simulink model "SingleTrackCANoe"  (R2021b)
settings: Solver=ode1  StartTime=0  StopTime=2  FixedStep=1.0000000000000000e-003  RelTol=1e-3
InitFcn:
  | sampleTime = str2double(get_param(bdroot, 'FixedStep'));
undefined symbols (not defined in the file or in its folder): AccPedalPos, BrakePedalPos, BrakeSwitch, DiscIntNeverNeededParam, DYNA4, EngSpd, IgnitionSwitch, InitialGear, InitialSpeed, IntendedEngTrq, LeftIndicator, MainBrakePress, MaxGear, MDL, MinGear, RefAcc, RefLane, RefLatPos, RefPath, RefPathCurv, RefSpd, RefSpdPreview, RefSpdRetrospect, RightIndicator, SteeringWheelAng, SteeringWheelTrq, UserDefinedRefValue, vm_const
libraries: UtilitiesLibrary x62, simulink x18, WheelSystemModules x14, LongitudinalControllerModules x13, LateralControllerModules x7, AnimationBusselectorModules x5, EnvironmentModules x5, BasicEngineControlModules x5, MiscellaneousControlModules x5, Animation3Modules x4, AuxiliariesModules x4, ReducedTireModules x4
(part 20 of 34)

== system SingleTrackCANoe/SimulationModel/Vehicle/Drivetrain/DrivetrainPhysics/DrivetrainPhysicsOutputs ==
  EngStates : Inport
  ClutchStates : Inport  Port=2
  TransmissionStates : Inport  Port=3
  TransferCase : Inport  Port=4
  FrontDifferentialStates : Inport  Port=5
  RearDifferentialStates : Inport  Port=6
  FrontLeftDifferentialStates : Inport  Port=7
  FrontRightDifferentialStates : Inport  Port=8
  RearLeftDifferentialStates : Inport  Port=9
  RearRightDifferentialStates : Inport  Port=10
  OutputDriveRatio : Inport  Port=11
  Bus Creator : BusCreator  Inputs=1
  Bus Creator4 : BusCreator  Inputs=2
  Bus Selector : BusSelector  OutputSignals=Physics.InSpd[rad/s],Physics.InAcc[rad/s**2]
  Bus Selector2 : BusSelector  OutputSignals=TrqDistributionFac[0_1]
  ClutchOutput : Subsystem
  Create TotalRatio/DrivetrainStates : DrivetrainModules/Create TotalRatio//DrivetrainStates  SystemSampleTime=-1  VariantActivationTime=update diagram  Latency=0  AutoFrameSizeCalculation=off
  DrivetrainPhysicsOutput : Subsystem  Tag=TESIS DYNAware Interface Block  mask{NeedsUpdate=off, SignalInfo=|}
      mask SignalInfo=|
      | {
      |   "Version": "4.6",
      |   "MuxedOutputBusName": "DrivetrainPhysics",
      |   "MuxedInputBusName": "input",
      |   "MuxedInputSelected": false,
      |   "MuxedOutputSelected": true,
      |   "SignalData": [
      |     {
      |       "initialValue": "0.0",
      |       "name": "EngSpd[rad/s]",
      |       "comment": "",
      |       "minString": "",
      |       "maxString": "",
      |       "width": 1,
      |       "dataType": 0,
      |       "signalType": 0,
      |       "createSignal": false,
      |       "outputName": "EngSpd[rad/s]",
      |       "generateSignalAccessBlock": false,
      |       "accessId": "$(parentId).$(blockName).$(outputName)"
      |     },
      |     {
      |       "initialValue": "0.0",
      |       "name": "EngAcc[rad/s**2]",
      |       "comment": "",
      |       "minString": "",
      |       "maxString": "",
      |       "width": 1,
      |       "dataType": 0,
      |       "signalType": 0,
      |       "createSignal": false,
      |       "outputName": "EngAcc[rad/s**2]",
      |       "generateSignalAccessBlock": false,
      |       "accessId": "$(parentId).$(blockName).$(outputName)"
      |     },
      |     {
      |       "initialValue": "0.0",
      |       "name": "Clutch",
      |       "comment": "",
      |       "minString": "",
      |       "maxString": "",
      |       "width": -1,
      |       "dataType": 0,
      |       "signalType": 1,
      |       "createSignal": false,
      |       "outputName": "Clutch",
      |       "generateSignalAccessBlock": false,
      |       "accessId": "$(parentId).$(blockName).$(outputName)"
      |     },
      |     {
      |       "initialValue": "0.0",
      |       "name": "Transmission",
      |       "comment": "",
      |       "minString": "",
      |       "maxString": "",
      |       "width": -1,
      |       "dataType": 0,
      |       "signalType": 1,
      |       "createSignal": false,
      |       "outputName": "Transmission",
      |       "generateSignalAccessBlock": false,
      |       "accessId": "$(parentId).$(blockName).$(outputName)"
      |     },
      |     {
      |       "initialValue": "0.0",
      |       "name": "TransferCase",
      |       "comment": "",
      |       "minString": "",
      |       "maxString": "",
      |       "width": -1,
      |       "dataType": 0,
      |       "signalType": 1,
      |       "createSignal": false,
      |       "outputName": "TransferCase",
      |       "generateSignalAccessBlock": false,
      |       "accessId": "$(parentId).$(blockName).$(outputName)"
      |     },
      |     {
      |       "initialValue": "0.0",
      |       "name": "FrontDifferential",
      |       "comment": "",
      |       "minString": "",
      |       "maxString": "",
      |       "width": -1,
      |       "dataType": 0,
      |       "signalType": 1,
      |       "createSignal": false,
      |       "outputName": "FrontDifferential",
      |       "generateSignalAccessBlock": false,
      |       "accessId": "$(parentId).$(blockName).$(outputName)"
      |     },
      |     {
      |       "initialValue": "0.0",
      |       "name": "FrontLeftShaft",
      |       "comment": "",
      |       "minString": "",
      |       "maxString": "",
      |       "width": -1,
      |       "dataType": 0,
      |       "signalType": 1,
      |       "createSignal": false,
      |       "outputName": "FrontLeftShaft",
      |       "generateSignalAccessBlock": false,
      |       "accessId": "$(parentId).$(blockName).$(outputName)"
      |     },
      |     {
      |       "initialValue": "0.0",
      |       "name": "FrontRightShaft",
      |       "comment": "",
      |       "minString": "",
      |       "maxString": "",
      |       "width": -1,
      |       "dataType": 0,
      |       "signalType": 1,
      |       "createSignal": false,
      |       "outputName": "FrontRightShaft",
      |       "generateSignalAccessBlock": false,
      |       "accessId": "$(parentId).$(blockName).$(outputName)"
      |     },
      |     {
      |       "initialValue": "0.0",
      |       "name": "RearDifferential",
      |       "comment": "",
      |       "minString": "",
      |       "maxString": "",
      |       "width": -1,
      |       "dataType": 0,
      |       "signalType": 1,
      |       "createSignal": false,
      |       "outputName": "RearDifferential",
      |       "generateSignalAccessBlock": false,
      |       "accessId": "$(parentId).$(blockName).$(outputName)"
      |     },
      |     {
      |       "initialValue": "0.0",
      |       "name": "RearLeftShaft",
      |       "comment": "",
      |       "minString": "",
      |       "maxString": "",
      |       "width": -1,
      |       "dataType": 0,
      |       "signalType": 1,
      |       "createSignal": false,
      |       "outputName": "RearLeftShaft",
      |       "generateSignalAccessBlock": false,
      |       "accessId": "$(parentId).$(blockName).$(outputName)"
      |     },
      |     {
      |       "initialValue": "0.0",
      |       "name": "RearRightShaft",
      |       "comment": "",
      |       "minString": "",
      |       "maxString": "",
      |       "width": -1,
      |       "dataType": 0,
      |       "signalType": 1,
      |       "createSignal": false,
      |       "outputName": "RearRightShaft",
      |       "generateSignalAccessBlock": false,
      |       "accessId": "$(parentId).$(blockName).$(outputName)"
      |     },
      |     {
      |       "initialValue": "0.0",
      |       "name": "Rear2LeftShaft",
      |       "comment": "",
      |       "minString": "",
      |       "maxString": "",
      |       "width": -1,
      |       "dataType": 0,
      |       "signalType": 1,
      |       "createSignal": false,
      |       "outputName": "Rear2LeftShaft",
      |       "generateSignalAccessBlock": false,
      |       "accessId": "$(parentId).$(blockName).$(outputName)"
      |     },
      |     {
      |       "initialValue": "0.0",
      |       "name": "Rear2RightShaft",
      |       "comment": "",
      |       "minString": "",
      |       "maxString": "",
      |       "width": -1,
      |       "dataType": 0,
      |       "signalType": 1,
      |       "createSignal": false,
      |       "outputName": "Rear2RightShaft",
      |       "generateSignalAccessBlock": false,
      |       "accessId": "$(parentId).$(blockName).$(outputName)"
      |     },
      |     {
      |       "initialValue": "0.0",
      |       "name": "Rear3LeftShaft",
      |       "comment": "",
      |       "minString": "",
      |       "maxString": "",
      |       "width": -1,
      |       "dataType": 0,
      |       "signalType": 1,
      |       "createSignal": false,
      |       "outputName": "Rear3LeftShaft",
      |       "generateSignalAccessBlock": false,
      |       "accessId": "$(parentId).$(blockName).$(outputName)"
      |     },
      |     {
      |       "initialValue": "0.0",
      |       "name": "Rear3RightShaft",
      |       "comment": "",
      |       "minString": "",
      |       "maxString": "",
      |       "width": -1,
      |       "dataType": 0,
      |       "signalType": 1,
      |       "createSignal": false,
      |       "outputName": "Rear3RightShaft",
      |       "generateSignalAccessBlock": false,
      |       "accessId": "$(parentId).$(blockName).$(outputName)"
      |     },
      |     {
      |       "initialValue": "0.0",
      |       "name": "TotalRatio[-]",
      |       "comment": "",
      |       "minString": "",
      |       "maxString": "",
      |       "width": 1,
      |       "dataType": 0,
      |       "signalType": 0,
      |       "createSignal": false,
      |       "outputName": "TotalRatio[-]",
      |       "generateSignalAccessBlock": false,
      |       "accessId": "$(parentId).$(blockName).$(outputName)"
      |     },
      |     {
      |       "initialValue": "0.0",
      |       "name": "DrivetrainStates",
      |       "comment": "",
      |       "minString": "",
      |       "maxString": "",
      |       "width": -1,
      |       "dataType": 0,
      |       "signalType": 1,
      |       "createSignal": false,
      |       "outputName": "DrivetrainStates",
      |       "generateSignalAccessBlock": false,
      |       "accessId": "$(parentId).$(blockName).$(outputName)"
      |     }
      |   ]
      | }
      mask prompts: NeedsUpdate "Specify, if subsystem content needs to be updated"; SignalInfo "Signal Info (json)"
      mask help: DYNA4 Interface Block Version 4.6
      mask init:
      | blockName = get_param(gcbh, 'Name');
      | parentId = DYNA4.ModelHandling.AccessID.getFromHierarchy(gcbh);
      | TD.InterfaceBlock.ModelCallbacks.GenerateContent(gcb);
      settings: DeleteFcn=TD.InterfaceBlock.ModelCallbacks.CloseGUI( gcbh );  NameChangeFcn=TD.InterfaceBlock.ModelCallbacks.BlockRenamedHandler(gcbh);  OpenFcn=TD.InterfaceBlock.ModelCallbacks.OpenGUI( gcbh );  CloseFcn=TD.InterfaceBlock.ModelCallbacks.CloseGUI( gcbh );
      mask Display:
      | image('InterfaceBlock.png','center');
      | port_label('input',1, 'EngSpd[rad/s]');
      | port_label('input',2, 'EngAcc[rad/s**2]');
      | port_label('input',3, 'Clutch');
      | port_label('input',4, 'Transmission');
      | port_label('input',5, 'TransferCase');
      | port_label('input',6, 'FrontDifferential');
      | port_label('input',7, 'FrontLeftShaft');
      | port_label('input',8, 'FrontRightShaft');
      | port_label('input',9, 'RearDifferential');
      | port_label('input',10, 'RearLeftShaft');
      | port_label('input',11, 'RearRightShaft');
      | port_label('input',12, 'Rear2LeftShaft');
      | port_label('input',13, 'Rear2RightShaft');
      | port_label('input',14, 'Rear3LeftShaft');
      | port_label('input',15, 'Rear3RightShaft');
      | port_label('input',16, 'TotalRatio[-]');
      | port_label('input',17, 'DrivetrainStates');
      | port_label('output',1, 'DrivetrainPhysics');
  FrontDifferentialOutput : Subsystem
  FrontLeftShaftOutput : Subsystem
  FrontRightShaftOutput : Subsystem
  PassThroughRatio : Constant
  Rear2LeftShaftOutput : Subsystem  Tag=TESIS DYNAware Interface Block  mask{NeedsUpdate=off, SignalInfo=|}
      mask SignalInfo=|
      | {
      |   "Version": "4.6",
      |   "MuxedOutputBusName": "Rear2LeftShaft",
      |   "MuxedInputBusName": "input",
      |   "MuxedInputSelected": false,
      |   "MuxedOutputSelected": true,
      |   "SignalData": [
      |     {
      |       "initialValue": "0.0",
      |       "name": "",
      |       "comment": "",
      |       "minString": "",
      |       "maxString": "",
      |       "width": 1,
      |       "dataType": 0,
      |       "signalType": 0,
      |       "createSignal": true,
      |       "outputName": "Trq[Nm]",
      |       "generateSignalAccessBlock": false,
      |       "accessId": "$(parentId).$(blockName).$(outputName)"
      |     },
      |     {
      |       "initialValue": "0.0",
      |       "name": "",
      |       "comment": "",
      |       "minString": "",
      |       "maxString": "",
      |       "width": 1,
      |       "dataType": 0,
      |       "signalType": 0,
      |       "createSignal": true,
      |       "outputName": "RotSpdDifferentialOut[rad/s]",
      |       "generateSignalAccessBlock": false,
      |       "accessId": "$(parentId).$(blockName).$(outputName)"
      |     },
      |     {
      |       "initialValue": "0.0",
      |       "name": "",
      |       "comment": "",
      |       "minString": "",
      |       "maxString": "",
      |       "width": 1,
      |       "dataType": 0,
      |       "signalType": 0,
      |       "createSignal": true,
      |       "outputName": "RotAcc[rad/s**2]",
      |       "generateSignalAccessBlock": false,
      |       "accessId": "$(parentId).$(blockName).$(outputName)"
      |     },
      |     {
      |       "initialValue": "0.0",
      |       "name": "",
      |       "comment": "",
      |       "minString": "",
      |       "maxString": "",
      |       "width": 1,
      |       "dataType": 0,
      |       "signalType": 0,
      |       "createSignal": true,
      |       "outputName": "DerivativeOfTrq_wrt_RotAng[Nm/rad]",
      |       "generateSignalAccessBlock": false,
      |       "accessId": "$(parentId).$(blockName).$(outputName)"
      |     },
      |     {
      |       "initialValue": "0.0",
      |       "name": "",
      |       "comment": "",
      |       "minString": "",
      |       "maxString": "",
      |       "width": 1,
      |       "dataType": 0,
      |       "signalType": 0,
      |       "createSignal": true,
      |       "outputName": "DerivativeOfTrq_wrt_WheelSpd[Nm/(rad/s)]",
      |       "generateSignalAccessBlock": false,
      |       "accessId": "$(parentId).$(blockName).$(outputName)"
      |     },
      |     {
      |       "initialValue": "0.0",
      |       "name": "",
      |       "comment": "",
      |       "minString": "",
      |       "maxString": "",
      |       "width": 1,
      |       "dataType": 0,
      |       "signalType": 0,
      |       "createSignal": true,
      |       "outputName": "AddInrt[kg*m**2]",
      |       "generateSignalAccessBlock": false,
      |       "accessId": "$(parentId).$(blockName).$(outputName)"
      |     },
      |     {
      |       "initialValue": "0.0",
      |       "name": "",
      |       "comment": "",
      |       "minString": "",
      |       "maxString": "",
      |       "width": 1,
      |       "dataType": 0,
      |       "signalType": 0,
      |       "createSignal": true,
      |       "outputName": "FrictionTrq[Nm]",
      |       "generateSignalAccessBlock": false,
      |       "accessId": "$(parentId).$(blockName).$(outputName)"
      |     }
      |   ]
      | }
      mask prompts: NeedsUpdate "Specify, if subsystem content needs to be updated"; SignalInfo "Signal Info (json)"
      mask help: DYNA4 Interface Block Version 4.6
      mask init:
      | blockName = get_param(gcbh, 'Name');
      | parentId = DYNA4.ModelHandling.AccessID.getFromHierarchy(gcbh);
      | TD.InterfaceBlock.ModelCallbacks.GenerateContent(gcb);
      settings: DeleteFcn=TD.InterfaceBlock.ModelCallbacks.CloseGUI( gcbh );  NameChangeFcn=TD.InterfaceBlock.ModelCallbacks.BlockRenamedHandler(gcbh);  OpenFcn=TD.InterfaceBlock.ModelCallbacks.OpenGUI( gcbh );  CloseFcn=TD.InterfaceBlock.ModelCallbacks.CloseGUI( gcbh );
      settings: AttributesFormatString=|
      | Trq[Nm] = 0.0
      | RotSpdDifferentialOut[rad/s] = 0.0
      | RotAcc[rad/s**2] = 0.0
      | DerivativeOfTrq_wrt_RotAng[Nm/rad] = 0.0
      | ...
      mask Display:
      | image('InterfaceBlock.png','center');
      | port_label('output',1, 'Rear2LeftShaft');
  Rear2RightShaftOutput : Subsystem  Tag=TESIS DYNAware Interface Block  mask{NeedsUpdate=off, SignalInfo=|}
      mask SignalInfo=|
      | {
      |   "Version": "4.6",
      |   "MuxedOutputBusName": "Rear2RightShaft",
      |   "MuxedInputBusName": "",
      |   "MuxedInputSelected": false,
      |   "MuxedOutputSelected": true,
      |   "SignalData": [
      |     {
      |       "initialValue": "0.0",
      |       "name": "",
      |       "comment": "",
      |       "minString": "",
      |       "maxString": "",
      |       "width": 1,
      |       "dataType": 0,
      |       "signalType": 0,
      |       "createSignal": true,
      |       "outputName": "Trq[Nm]",
      |       "generateSignalAccessBlock": false,
      |       "accessId": "$(parentId).$(blockName).$(outputName)"
      |     },
      |     {
      |       "initialValue": "0.0",
      |       "name": "",
      |       "comment": "",
      |       "minString": "",
      |       "maxString": "",
      |       "width": 1,
      |       "dataType": 0,
      |       "signalType": 0,
      |       "createSignal": true,
      |       "outputName": "RotSpdDifferentialOut[rad/s]",
      |       "generateSignalAccessBlock": false,
      |       "accessId": "$(parentId).$(blockName).$(outputName)"
      |     },
      |     {
      |       "initialValue": "0.0",
      |       "name": "",
      |       "comment": "",
      |       "minString": "",
      |       "maxString": "",
      |       "width": 1,
      |       "dataType": 0,
      |       "signalType": 0,
      |       "createSignal": true,
      |       "outputName": "RotAcc[rad/s**2]",
      |       "generateSignalAccessBlock": false,
      |       "accessId": "$(parentId).$(blockName).$(outputName)"
      |     },
      |     {
      |       "initialValue": "0.0",
      |       "name": "",
      |       "comment": "",
      |       "minString": "",
      |       "maxString": "",
      |       "width": 1,
      |       "dataType": 0,
      |       "signalType": 0,
      |       "createSignal": true,
      |       "outputName": "DerivativeOfTrq_wrt_RotAng[Nm/rad]",
      |       "generateSignalAccessBlock": false,
      |       "accessId": "$(parentId).$(blockName).$(outputName)"
      |     },
      |     {
      |       "initialValue": "0.0",
      |       "name": "",
      |       "comment": "",
      |       "minString": "",
      |       "maxString": "",
      |       "width": 1,
      |       "dataType": 0,
      |       "signalType": 0,
      |       "createSignal": true,
      |       "outputName": "DerivativeOfTrq_wrt_WheelSpd[Nm/(rad/s)]",
      |       "generateSignalAccessBlock": false,
      |       "accessId": "$(parentId).$(blockName).$(outputName)"
      |     },
      |     {
      |       "initialValue": "0.0",
      |       "name": "",
      |       "comment": "",
      |       "minString": "",
      |       "maxString": "",
      |       "width": 1,
      |       "dataType": 0,
      |       "signalType": 0,
      |       "createSignal": true,
      |       "outputName": "AddInrt[kg*m**2]",
      |       "generateSignalAccessBlock": false,
      |       "accessId": "$(parentId).$(blockName).$(outputName)"
      |     },
      |     {
      |       "initialValue": "0.0",
      |       "name": "",
      |       "comment": "",
      |       "minString": "",
      |       "maxString": "",
      |       "width": 1,
      |       "dataType": 0,
      |       "signalType": 0,
      |       "createSignal": true,
      |       "outputName": "FrictionTrq[Nm]",
      |       "generateSignalAccessBlock": false,
      |       "accessId": "$(parentId).$(blockName).$(outputName)"
      |     }
      |   ]
      | }
      mask prompts: NeedsUpdate "Specify, if subsystem content needs to be updated"; SignalInfo "Signal Info (json)"
      mask help: DYNA4 Interface Block Version 4.6
      mask init:
      | blockName = get_param(gcbh, 'Name');
      | parentId = DYNA4.ModelHandling.AccessID.getFromHierarchy(gcbh);
      | TD.InterfaceBlock.ModelCallbacks.GenerateContent(gcb);
      settings: DeleteFcn=TD.InterfaceBlock.ModelCallbacks.CloseGUI( gcbh );  NameChangeFcn=TD.InterfaceBlock.ModelCallbacks.BlockRenamedHandler(gcbh);  OpenFcn=TD.InterfaceBlock.ModelCallbacks.OpenGUI( gcbh );  CloseFcn=TD.InterfaceBlock.ModelCallbacks.CloseGUI( gcbh );
      settings: AttributesFormatString=|
      | Trq[Nm] = 0.0
      | RotSpdDifferentialOut[rad/s] = 0.0
      | RotAcc[rad/s**2] = 0.0
      | DerivativeOfTrq_wrt_RotAng[Nm/rad] = 0.0
      | ...
      mask Display:
      | image('InterfaceBlock.png','center');
      | port_label('output',1, 'Rear2RightShaft');
  Rear3LeftShaftOutput : Subsystem  Tag=TESIS DYNAware Interface Block  mask{NeedsUpdate=off, SignalInfo=|}
      mask SignalInfo=|
      | {
      |   "Version": "4.6",
      |   "MuxedOutputBusName": "Rear3LeftShaft",
      |   "MuxedInputBusName": "",
      |   "MuxedInputSelected": false,
      |   "MuxedOutputSelected": true,
      |   "SignalData": [
      |     {
      |       "initialValue": "0.0",
      |       "name": "",
      |       "comment": "",
      |       "minString": "",
      |       "maxString": "",
      |       "width": 1,
      |       "dataType": 0,
      |       "signalType": 0,
      |       "createSignal": true,
      |       "outputName": "Trq[Nm]",
      |       "generateSignalAccessBlock": false,
      |       "accessId": "$(parentId).$(blockName).$(outputName)"
      |     },
      |     {
      |       "initialValue": "0.0",
      |       "name": "",
      |       "comment": "",
      |       "minString": "",
      |       "maxString": "",
      |       "width": 1,
      |       "dataType": 0,
      |       "signalType": 0,
      |       "createSignal": true,
      |       "outputName": "RotSpdDifferentialOut[rad/s]",
      |       "generateSignalAccessBlock": false,
      |       "accessId": "$(parentId).$(blockName).$(outputName)"
      |     },
      |     {
      |       "initialValue": "0.0",
      |       "name": "",
      |       "comment": "",
      |       "minString": "",
      |       "maxString": "",
      |       "width": 1,
      |       "dataType": 0,
      |       "signalType": 0,
      |       "createSignal": true,
      |       "outputName": "RotAcc[rad/s**2]",
      |       "generateSignalAccessBlock": false,
      |       "accessId": "$(parentId).$(blockName).$(outputName)"
      |     },
      |     {
      |       "initialValue": "0.0",
      |       "name": "",
      |       "comment": "",
      |       "minString": "",
      |       "maxString": "",
      |       "width": 1,
      |       "dataType": 0,
      |       "signalType": 0,
      |       "createSignal": true,
      |       "outputName": "DerivativeOfTrq_wrt_RotAng[Nm/rad]",
      |       "generateSignalAccessBlock": false,
      |       "accessId": "$(parentId).$(blockName).$(outputName)"
      |     },
      |     {
      |       "initialValue": "0.0",
      |       "name": "",
      |       "comment": "",
      |       "minString": "",
      |       "maxString": "",
      |       "width": 1,
      |       "dataType": 0,
      |       "signalType": 0,
      |       "createSignal": true,
      |       "outputName": "DerivativeOfTrq_wrt_WheelSpd[Nm/(rad/s)]",
      |       "generateSignalAccessBlock": false,
      |       "accessId": "$(parentId).$(blockName).$(outputName)"
      |     },
      |     {
      |       "initialValue": "0.0",
      |       "name": "",
      |       "comment": "",
      |       "minString": "",
      |       "maxString": "",
      |       "width": 1,
      |       "dataType": 0,
      |       "signalType": 0,
      |       "createSignal": true,
      |       "outputName": "AddInrt[kg*m**2]",
      |       "generateSignalAccessBlock": false,
      |       "accessId": "$(parentId).$(blockName).$(outputName)"
      |     },
      |     {
      |       "initialValue": "0.0",
      |       "name": "",
      |       "comment": "",
      |       "minString": "",
      |       "maxString": "",
      |       "width": 1,
      |       "dataType": 0,
      |       "signalType": 0,
      |       "createSignal": true,
      |       "outputName": "FrictionTrq[Nm]",
      |       "generateSignalAccessBlock": false,
      |       "accessId": "$(parentId).$(blockName).$(outputName)"
      |     }
      |   ]
      | }
      mask prompts: NeedsUpdate "Specify, if subsystem content needs to be updated"; SignalInfo "Signal Info (json)"
      mask help: DYNA4 Interface Block Version 4.6
      mask init:
      | blockName = get_param(gcbh, 'Name');
      | parentId = DYNA4.ModelHandling.AccessID.getFromHierarchy(gcbh);
      | TD.InterfaceBlock.ModelCallbacks.GenerateContent(gcb);
      settings: DeleteFcn=TD.InterfaceBlock.ModelCallbacks.CloseGUI( gcbh );  NameChangeFcn=TD.InterfaceBlock.ModelCallbacks.BlockRenamedHandler(gcbh);  OpenFcn=TD.InterfaceBlock.ModelCallbacks.OpenGUI( gcbh );  CloseFcn=TD.InterfaceBlock.ModelCallbacks.CloseGUI( gcbh );
      settings: AttributesFormatString=|
      | Trq[Nm] = 0.0
      | RotSpdDifferentialOut[rad/s] = 0.0
      | RotAcc[rad/s**2] = 0.0
      | DerivativeOfTrq_wrt_RotAng[Nm/rad] = 0.0
      | ...
      mask Display:
      | image('InterfaceBlock.png','center');
      | port_label('output',1, 'Rear3LeftShaft');
  Rear3RightShaftOutput : Subsystem  Tag=TESIS DYNAware Interface Block  mask{NeedsUpdate=off, SignalInfo=|}
      mask SignalInfo=|
      | {
      |   "Version": "4.6",
      |   "MuxedOutputBusName": "Rear3RightShaft",
      |   "MuxedInputBusName": "",
      |   "MuxedInputSelected": false,
      |   "MuxedOutputSelected": true,
      |   "SignalData": [
      |     {
      |       "initialValue": "0.0",
      |       "name": "",
      |       "comment": "",
      |       "minString": "",
      |       "maxString": "",
      |       "width": 1,
      |       "dataType": 0,
      |       "signalType": 0,
      |       "createSignal": true,
      |       "outputName": "Trq[Nm]",
      |       "generateSignalAccessBlock": false,
      |       "accessId": "$(parentId).$(blockName).$(outputName)"
      |     },
      |     {
      |       "initialValue": "0.0",
      |       "name": "",
      |       "comment": "",
      |       "minString": "",
      |       "maxString": "",
      |       "width": 1,
      |       "dataType": 0,
      |       "signalType": 0,
      |       "createSignal": true,
      |       "outputName": "RotSpdDifferentialOut[rad/s]",
      |       "generateSignalAccessBlock": false,
      |       "accessId": "$(parentId).$(blockName).$(outputName)"
      |     },
      |     {
      |       "initialValue": "0.0",
      |       "name": "",
      |       "comment": "",
      |       "minString": "",
      |       "maxString": "",
      |       "width": 1,
      |       "dataType": 0,
      |       "signalType": 0,
      |       "createSignal": true,
      |       "outputName": "RotAcc[rad/s**2]",
      |       "generateSignalAccessBlock": false,
      |       "accessId": "$(parentId).$(blockName).$(outputName)"
      |     },
      |     {
      |       "initialValue": "0.0",
      |       "name": "",
      |       "comment": "",
      |       "minString": "",
      |       "maxString": "",
      |       "width": 1,
      |       "dataType": 0,
      |       "signalType": 0,
      |       "createSignal": true,
      |       "outputName": "DerivativeOfTrq_wrt_RotAng[Nm/rad]",
      |       "generateSignalAccessBlock": false,
      |       "accessId": "$(parentId).$(blockName).$(outputName)"
      |     },
      |     {
      |       "initialValue": "0.0",
      |       "name": "",
      |       "comment": "",
      |       "minString": "",
      |       "maxString": "",
      |       "width": 1,
      |       "dataType": 0,
      |       "signalType": 0,
      |       "createSignal": true,
      |       "outputName": "DerivativeOfTrq_wrt_WheelSpd[Nm/(rad/s)]",
      |       "generateSignalAccessBlock": false,
      |       "accessId": "$(parentId).$(blockName).$(outputName)"
      |     },
      |     {
      |       "initialValue": "0.0",
      |       "name": "",
      |       "comment": "",
      |       "minString": "",
      |       "maxString": "",
      |       "width": 1,
      |       "dataType": 0,
      |       "signalType": 0,
      |       "createSignal": true,
      |       "outputName": "AddInrt[kg*m**2]",
      |       "generateSignalAccessBlock": false,
      |       "accessId": "$(parentId).$(blockName).$(outputName)"
      |     },
      |     {
      |       "initialValue": "0.0",
      |       "name": "",
      |       "comment": "",
      |       "minString": "",
      |       "maxString": "",
      |       "width": 1,
      |       "dataType": 0,
      |       "signalType": 0,
      |       "createSignal": true,
      |       "outputName": "FrictionTrq[Nm]",
      |       "generateSignalAccessBlock": false,
      |       "accessId": "$(parentId).$(blockName).$(outputName)"
      |     }
      |   ]
      | }
      mask prompts: NeedsUpdate "Specify, if subsystem content needs to be updated"; SignalInfo "Signal Info (json)"
      mask help: DYNA4 Interface Block Version 4.6
      mask init:
      | blockName = get_param(gcbh, 'Name');
      | parentId = DYNA4.ModelHandling.AccessID.getFromHierarchy(gcbh);
      | TD.InterfaceBlock.ModelCallbacks.GenerateContent(gcb);
      settings: DeleteFcn=TD.InterfaceBlock.ModelCallbacks.CloseGUI( gcbh );  NameChangeFcn=TD.InterfaceBlock.ModelCallbacks.BlockRenamedHandler(gcbh);  OpenFcn=TD.InterfaceBlock.ModelCallbacks.OpenGUI( gcbh );  CloseFcn=TD.InterfaceBlock.ModelCallbacks.CloseGUI( gcbh );
      settings: AttributesFormatString=|
      | Trq[Nm] = 0.0
      | RotSpdDifferentialOut[rad/s] = 0.0
      | RotAcc[rad/s**2] = 0.0
      | DerivativeOfTrq_wrt_RotAng[Nm/rad] = 0.0
      | ...
      mask Display:
      | image('InterfaceBlock.png','center');
      | port_label('output',1, 'Rear3RightShaft');
  RearDifferentialOutput : Subsystem
  RearLeftShaftOutput : Subsystem
  RearRightShaftOutput : Subsystem
  Terminator : Terminator
  TotalRatio : Subsystem
  TransferCaseOutput : Subsystem
  TransmissionOutput : Subsystem
  DrivetrainPhysics : Outport  VectorParamsAs1DForOutWhenUnconnected=off
  wires:
  TransferCase/1 -> Bus Selector2/1, TransferCaseOutput/1(TransferCaseStates)
  TransmissionStates/1 -> TransmissionOutput/1(TransmissionStates), Create TotalRatio/DrivetrainStates/1, TotalRatio/1(TransmissionStates)
  EngStates/1 -> Bus Selector/1
  DrivetrainPhysicsOutput/1(DrivetrainPhysics___UNIQUE_1) -> DrivetrainPhysics/1
  ClutchOutput/1(Clutch) -> DrivetrainPhysicsOutput/3(Clutch___UNIQUE_1)
  TransmissionOutput/1(Transmission) -> DrivetrainPhysicsOutput/4(Transmission___UNIQUE_1)
  FrontLeftShaftOutput/1(FrontLeftShaft) -> DrivetrainPhysicsOutput/7(FrontLeftShaft___UNIQUE_1)
  FrontRightShaftOutput/1(FrontRightShaft) -> DrivetrainPhysicsOutput/8(FrontRightShaft___UNIQUE_1)
  RearRightShaftOutput/1(RearRightShaft) -> DrivetrainPhysicsOutput/11(RearRightShaft___UNIQUE_1)
  Rear2LeftShaftOutput/1(Rear2LeftShaft___UNIQUE_1) -> DrivetrainPhysicsOutput/12(Rear2LeftShaft___UNIQUE_1)
  Rear2RightShaftOutput/1(Rear2RightShaft___UNIQUE_1) -> DrivetrainPhysicsOutput/13(Rear2RightShaft___UNIQUE_1)
  Rear3LeftShaftOutput/1(Rear3LeftShaft___UNIQUE_1) -> DrivetrainPhysicsOutput/14(Rear3LeftShaft___UNIQUE_1)
  Rear3RightShaftOutput/1(Rear3RightShaft___UNIQUE_1) -> DrivetrainPhysicsOutput/15(Rear3RightShaft___UNIQUE_1)
  TotalRatio/1(TotalRatio) -> DrivetrainPhysicsOutput/16(TotalRatio[-]___UNIQUE_1)
  ClutchStates/1 -> ClutchOutput/1(ClutchStates)
  RearLeftShaftOutput/1(RearLeftShaft) -> DrivetrainPhysicsOutput/10(RearLeftShaft___UNIQUE_1)
  FrontDifferentialStates/1 -> FrontDifferentialOutput/1(FrontDifferentialStates)
  RearDifferentialStates/1 -> RearDifferentialOutput/1(RearDifferentialStates)
  RearLeftDifferentialStates/1 -> RearLeftShaftOutput/1(In1)
  RearRightDifferentialStates/1 -> RearRightShaftOutput/1(In1)
  FrontLeftDifferentialStates/1 -> FrontLeftShaftOutput/1(In1)
  FrontRightDifferentialStates/1 -> FrontRightShaftOutput/1(In1)
  Bus Selector/1 -> DrivetrainPhysicsOutput/1(EngSpd[rad/s]___UNIQUE_1)  "<InSpd[rad/s]>"
  Bus Selector/2 -> DrivetrainPhysicsOutput/2(EngAcc[rad/s**2]___UNIQUE_1)  "<InAcc[rad/s**2]>"
  TransferCaseOutput/1(TransferCase) -> DrivetrainPhysicsOutput/5(TransferCase___UNIQUE_1)
  FrontDifferentialOutput/1(FrontDifferential) -> DrivetrainPhysicsOutput/6(FrontDifferential___UNIQUE_1)
  RearDifferentialOutput/1(RearDifferential) -> DrivetrainPhysicsOutput/9(RearDifferential___UNIQUE_1)
  OutputDriveRatio/1 -> TotalRatio/2(OutputDriveRatio)
  Create TotalRatio/DrivetrainStates/1 -> Terminator/1
  Create TotalRatio/DrivetrainStates/2 -> DrivetrainPhysicsOutput/17(DrivetrainStates___UNIQUE_1)
  Bus Creator/1 -> Create TotalRatio/DrivetrainStates/2  "Info"
  PassThroughRatio/1 -> Bus Creator/1, Bus Creator4/1  "Ratio[-]"
  Bus Selector2/1 -> Bus Creator4/2  "<TrqDistributionFac[0_1]>"
  Bus Creator4/1 -> Create TotalRatio/DrivetrainStates/3, Create TotalRatio/DrivetrainStates/4, Create TotalRatio/DrivetrainStates/5  "Info"

== system SingleTrackCANoe/SimulationModel/Vehicle/Drivetrain/DrivetrainPhysics/DynaComponentInfo ==

== system SingleTrackCANoe/SimulationModel/Vehicle/Engine/EngineControlUnit/DynaComponentInfo ==

== system SingleTrackCANoe/SimulationModel/Vehicle/Engine/EngineControlUnit/EngineControlUnitOutput ==
  StarterSwitch[0;1]___UNIQUE_1 : Inport  Description=|  PortDimensions=[1]
      | <name>StarterSwitch[0;1]</name>
      | <comment>Engine starter switch</comment>
  EngRunPermission[0;1]___UNIQUE_1 : Inport  Description=|  Port=2  PortDimensions=[1]
      | <name>EngRunPermission[0;1]</name>
      | <comment>Switch indicating a engine stop due to start stop function or ignition off</comment>
  EngLoadSignal[0_1]___UNIQUE_1 : Inport  Description=|  Port=3  PortDimensions=[1]
      | <name>EngLoadSignal[0_1]</name>
      | <comment>Engine load signal</comment>
  EngIdleSpd[rad/s]___UNIQUE_1 : Inport  Description=|  Port=4  PortDimensions=[1]
      | <name>EngIdleSpd[rad/s]</name>
      | <comment>Engine idle speed</comment>
  EngFuelCutoff[0;1]___UNIQUE_1 : Inport  Description=|  Port=5  PortDimensions=[1]
      | <name>EngFuelCutoff[0;1]</name>
      | <comment>Logical signal which is true if fuel mass flow is stopped</comment>
  MaxEngSpd[rad/s]___UNIQUE_1 : Inport  Description=|  Port=6  PortDimensions=[1]
      | <name>MaxEngSpd[rad/s]</name>
      | <comment>Maximum allowed engine speed, threshold for fuel cut off</comment>
  UpperEngTrqSwitch[0;2]___UNIQUE_1 : Inport  Description=|  Port=7  PortDimensions=[1]
      | <name>UpperEngTrqSwitch[0;2]</name>
      | <comment>Switch indicating how the upper engine torque should be restricted (0: off, 1: slow, 2: fast)</comment>
  UpperEngTrqLimit[Nm]___UNIQUE_1 : Inport  Description=|  Port=8  PortDimensions=[1]
      | <name>UpperEngTrqLimit[Nm]</name>
      | <comment>Upper limit for the engine torque</comment>
  LowerEngTrqSwitch[0;2]___UNIQUE_1 : Inport  Description=|  Port=9  PortDimensions=[1]
      | <name>LowerEngTrqSwitch[0;2]</name>
      | <comment>Switch indicating how the lower engine torque should be restricted (0: off, 1: slow, 2: fast)</comment>
  LowerEngTrqLimit[Nm]___UNIQUE_1 : Inport  Description=|  Port=10  PortDimensions=[1]
      | <name>LowerEngTrqLimit[Nm]</name>
      | <comment>Lower limit for the engine torque</comment>
  __TDD__EngineControlUnit.EngFuelCutoff[0;1] : Demux  Outputs=[1]
  __TDD__EngineControlUnit.EngIdleSpd[rad/s] : Demux  Outputs=[1]
  __TDD__EngineControlUnit.EngLoadSignal[0_1] : Demux  Outputs=[1]
  __TDD__EngineControlUnit.EngRunPermission[0;1] : Demux  Outputs=[1]
  __TDD__EngineControlUnit.LowerEngTrqLimit[Nm] : Demux  Outputs=[1]
  __TDD__EngineControlUnit.LowerEngTrqSwitch[0;2] : Demux  Outputs=[1]
  __TDD__EngineControlUnit.MaxEngSpd[rad/s] : Demux  Outputs=[1]
  __TDD__EngineControlUnit.StarterSwitch[0;1] : Demux  Outputs=[1]
  __TDD__EngineControlUnit.UpperEngTrqLimit[Nm] : Demux  Outputs=[1]
  __TDD__EngineControlUnit.UpperEngTrqSwitch[0;2] : Demux  Outputs=[1]
  __TDO__EngineControlUnit : BusCreator  Inputs=10
  EngineControlUnit___UNIQUE_1 : Outport  Description=|  PortDimensions=[10]  VectorParamsAs1DForOutWhenUnconnected=off
      | <name>StarterSwitch[0;1]</name>
      | <comment>Engine starter switch</comment>
  wires:
  __TDO__EngineControlUnit/1 -> EngineControlUnit___UNIQUE_1/1  "EngineControlUnit"
  __TDD__EngineControlUnit.LowerEngTrqLimit[Nm]/1 -> __TDO__EngineControlUnit/10  "LowerEngTrqLimit[Nm]"
  LowerEngTrqLimit[Nm]___UNIQUE_1/1 -> __TDD__EngineControlUnit.LowerEngTrqLimit[Nm]/1
  __TDD__EngineControlUnit.LowerEngTrqSwitch[0;2]/1 -> __TDO__EngineControlUnit/9  "LowerEngTrqSwitch[0;2]"
  LowerEngTrqSwitch[0;2]___UNIQUE_1/1 -> __TDD__EngineControlUnit.LowerEngTrqSwitch[0;2]/1
  __TDD__EngineControlUnit.UpperEngTrqLimit[Nm]/1 -> __TDO__EngineControlUnit/8  "UpperEngTrqLimit[Nm]"
  UpperEngTrqLimit[Nm]___UNIQUE_1/1 -> __TDD__EngineControlUnit.UpperEngTrqLimit[Nm]/1
  __TDD__EngineControlUnit.UpperEngTrqSwitch[0;2]/1 -> __TDO__EngineControlUnit/7  "UpperEngTrqSwitch[0;2]"
  UpperEngTrqSwitch[0;2]___UNIQUE_1/1 -> __TDD__EngineControlUnit.UpperEngTrqSwitch[0;2]/1
  __TDD__EngineControlUnit.MaxEngSpd[rad/s]/1 -> __TDO__EngineControlUnit/6  "MaxEngSpd[rad/s]"
  MaxEngSpd[rad/s]___UNIQUE_1/1 -> __TDD__EngineControlUnit.MaxEngSpd[rad/s]/1
  __TDD__EngineControlUnit.EngFuelCutoff[0;1]/1 -> __TDO__EngineControlUnit/5  "EngFuelCutoff[0;1]"
  EngFuelCutoff[0;1]___UNIQUE_1/1 -> __TDD__EngineControlUnit.EngFuelCutoff[0;1]/1
  __TDD__EngineControlUnit.EngIdleSpd[rad/s]/1 -> __TDO__EngineControlUnit/4  "EngIdleSpd[rad/s]"
  EngIdleSpd[rad/s]___UNIQUE_1/1 -> __TDD__EngineControlUnit.EngIdleSpd[rad/s]/1
  __TDD__EngineControlUnit.EngLoadSignal[0_1]/1 -> __TDO__EngineControlUnit/3  "EngLoadSignal[0_1]"
  EngLoadSignal[0_1]___UNIQUE_1/1 -> __TDD__EngineControlUnit.EngLoadSignal[0_1]/1
  __TDD__EngineControlUnit.EngRunPermission[0;1]/1 -> __TDO__EngineControlUnit/2  "EngRunPermission[0;1]"
  EngRunPermission[0;1]___UNIQUE_1/1 -> __TDD__EngineControlUnit.EngRunPermission[0;1]/1
  __TDD__EngineControlUnit.StarterSwitch[0;1]/1 -> __TDO__EngineControlUnit/1  "StarterSwitch[0;1]"
  StarterSwitch[0;1]___UNIQUE_1/1 -> __TDD__EngineControlUnit.StarterSwitch[0;1]/1

== system SingleTrackCANoe/SimulationModel/Vehicle/Engine/EngineControlUnit/InputFromCTRL ==
  fromCTRL : Inport
  TDBusSelector : BusSelector  OutputSignals=CTRL.LongitudinalControl.IgnitionSwitch[0;3],CTRL.LongitudinalControl.EngRunPermission[0;1],CTRL.LongitudinalControl.AccPedalPos[0_1],CTRL.LongitudinalControl.IntendedEngTrq[Nm],CTRL.LongitudinalControl.IntendedEngTrqActive[0;1],CTRL.LongitudinalControl.ClutchPos[0_1]
  __TDD__AccPedalPos[0_1] : Demux  Outputs=1
  __TDD__ClutchPos[0_1] : Demux  Outputs=[1]
  __TDD__EngRunPermission[0;1] : Demux  Outputs=[1]
  __TDD__IgnitionSwitch[0;3] : Demux  Outputs=[1]
  __TDD__IntendedEngTrqActive[0;1] : Demux  Outputs=[1]
  __TDD__IntendedEngTrq[Nm] : Demux  Outputs=[1]
  IgnitionSwitch[0;3]___UNIQUE_1 : Outport  Description=|  PortDimensions=[1]  VectorParamsAs1DForOutWhenUnconnected=off
      | <name>CTRL.LongitudinalControl.IgnitionSwitch[0;3]</name>
      | <comment>Ignition signal with four signal states: 0 - ignition off + consumer off + starter off, 1 - ignition off + consumer on + starter off, 2 - ignition on + consumer on + starter off, 3 - ignition on + consumer on  + starter on</comment>
  EngRunPermission[0;1]___UNIQUE_1 : Outport  Description=|  Port=2  PortDimensions=[1]  VectorParamsAs1DForOutWhenUnconnected=off
      | <name>CTRL.LongitudinalControl.EngRunPermission[0;1]</name>
      | <comment></comment>
  AccPedalPos[0_1]___UNIQUE_1 : Outport  Description=|  Port=3  VectorParamsAs1DForOutWhenUnconnected=off
      | <name>CTRL.LongitudinalControl.AccPedalPos[0_1]</name>
      | <comment></comment>
  IntendedEngTrq[Nm]___UNIQUE_1 : Outport  Description=|  Port=4  PortDimensions=[1]  VectorParamsAs1DForOutWhenUnconnected=off
      | <name>CTRL.LongitudinalControl.IntendedEngTrq[Nm]</name>
      | <comment></comment>
  IntendedEngTrqActive[0;1]___UNIQUE_1 : Outport  Description=|  Port=5  PortDimensions=[1]  VectorParamsAs1DForOutWhenUnconnected=off
      | <name>CTRL.LongitudinalControl.IntendedEngTrqActive[0;1]</name>
      | <comment></comment>
  ClutchPos[0_1]___UNIQUE_1 : Outport  Description=|  Port=6  PortDimensions=[1]  VectorParamsAs1DForOutWhenUnconnected=off
      | <name>CTRL.LongitudinalControl.ClutchPos[0_1]</name>
      | <comment>Clutch position</comment>
  wires:
  __TDD__ClutchPos[0_1]/1 -> ClutchPos[0_1]___UNIQUE_1/1  "ClutchPos[0_1]"
  __TDD__IntendedEngTrqActive[0;1]/1 -> IntendedEngTrqActive[0;1]___UNIQUE_1/1  "IntendedEngTrqActive[0;1]"
  __TDD__IntendedEngTrq[Nm]/1 -> IntendedEngTrq[Nm]___UNIQUE_1/1  "IntendedEngTrq[Nm]"
  __TDD__AccPedalPos[0_1]/1 -> AccPedalPos[0_1]___UNIQUE_1/1  "AccPedalPos[0_1]"
  __TDD__EngRunPermission[0;1]/1 -> EngRunPermission[0;1]___UNIQUE_1/1  "EngRunPermission[0;1]"
  __TDD__IgnitionSwitch[0;3]/1 -> IgnitionSwitch[0;3]___UNIQUE_1/1  "IgnitionSwitch[0;3]"
  TDBusSelector/6 -> __TDD__ClutchPos[0_1]/1  "<ClutchPos[0_1]>"
  TDBusSelector/5 -> __TDD__IntendedEngTrqActive[0;1]/1  "<IntendedEngTrqActive[0;1]>"
  TDBusSelector/4 -> __TDD__IntendedEngTrq[Nm]/1  "<IntendedEngTrq[Nm]>"
  TDBusSelector/3 -> __TDD__AccPedalPos[0_1]/1  "<AccPedalPos[0_1]>"
  TDBusSelector/2 -> __TDD__EngRunPermission[0;1]/1  "<EngRunPermission[0;1]>"
  TDBusSelector/1 -> __TDD__IgnitionSwitch[0;3]/1  "<IgnitionSwitch[0;3]>"
  fromCTRL/1 -> TDBusSelector/1

== system SingleTrackCANoe/SimulationModel/Vehicle/Engine/EngineControlUnit/InputFromCTRL1 ==
  fromCTRL : Inport
  TDBusSelector : BusSelector  OutputSignals=CTRL.LongitudinalControl.ASRRequestSwitch[0;2],CTRL.LongitudinalControl.ASRTrq[Nm],CTRL.LongitudinalControl.MSRRequestSwitch[0;2],CTRL.LongitudinalControl.MSRTrq[Nm]
  __TDD__ASRRequestSwitch[0;2] : Demux  Outputs=1
  __TDD__ASRTrq[Nm] : Demux  Outputs=1
  __TDD__MSRRequestSwitch[0;2] : Demux  Outputs=1
  __TDD__MSRTrq[Nm] : Demux  Outputs=1
  ASRRequestSwitch[0;2]___UNIQUE_1 : Outport  Description=|  VectorParamsAs1DForOutWhenUnconnected=off
      | <name>CTRL.LongitudinalControl.ASRRequestSwitch[0;2]</name>
      | <comment></comment>
  ASRTrq[Nm]___UNIQUE_1 : Outport  Description=|  Port=2  VectorParamsAs1DForOutWhenUnconnected=off
      | <name>CTRL.LongitudinalControl.ASRTrq[Nm]</name>
      | <comment></comment>
  MSRRequestSwitch[0;2]___UNIQUE_1 : Outport  Description=|  Port=3  VectorParamsAs1DForOutWhenUnconnected=off
      | <name>CTRL.LongitudinalControl.MSRRequestSwitch[0;2]</name>
      | <comment></comment>
  MSRTrq[Nm]___UNIQUE_1 : Outport  Description=|  Port=4  VectorParamsAs1DForOutWhenUnconnected=off
      | <name>CTRL.LongitudinalControl.MSRTrq[Nm]</name>
      | <comment></comment>
  wires:
  __TDD__MSRTrq[Nm]/1 -> MSRTrq[Nm]___UNIQUE_1/1  "MSRTrq[Nm]"
  __TDD__MSRRequestSwitch[0;2]/1 -> MSRRequestSwitch[0;2]___UNIQUE_1/1  "MSRRequestSwitch[0;2]"
  __TDD__ASRTrq[Nm]/1 -> ASRTrq[Nm]___UNIQUE_1/1  "ASRTrq[Nm]"
  __TDD__ASRRequestSwitch[0;2]/1 -> ASRRequestSwitch[0;2]___UNIQUE_1/1  "ASRRequestSwitch[0;2]"
  TDBusSelector/4 -> __TDD__MSRTrq[Nm]/1  "<MSRTrq[Nm]>"
  TDBusSelector/3 -> __TDD__MSRRequestSwitch[0;2]/1  "<MSRRequestSwitch[0;2]>"
  TDBusSelector/2 -> __TDD__ASRTrq[Nm]/1  "<ASRTrq[Nm]>"
  TDBusSelector/1 -> __TDD__ASRRequestSwitch[0;2]/1  "<ASRRequestSwitch[0;2]>"
  fromCTRL/1 -> TDBusSelector/1

== system SingleTrackCANoe/SimulationModel/Vehicle/Engine/EngineControlUnit/InputFromChassis ==
  fromChassis : Inport
  TDBusSelector : BusSelector  OutputSignals=VehicleBody.AbsVel[m/s]
  __TDD__AbsVel[m/s] : Demux  Outputs=1
  AbsVel[m/s]___UNIQUE_1 : Outport  Description=|  VectorParamsAs1DForOutWhenUnconnected=off
      | <name>VehicleBody.AbsVel[m/s]</name>
      | <comment></comment>
  wires:
  __TDD__AbsVel[m/s]/1 -> AbsVel[m/s]___UNIQUE_1/1  "AbsVel[m/s]"
  TDBusSelector/1 -> __TDD__AbsVel[m/s]/1  "<AbsVel[m/s]>"
  fromChassis/1 -> TDBusSelector/1

== system SingleTrackCANoe/SimulationModel/Vehicle/Engine/EngineControlUnit/InputFromDrivetrain ==
  fromDrivetrain : Inport
  TDBusSelector : BusSelector  OutputSignals=DrivetrainPhysics.Transmission.Gear[-4;20],DrivetrainPhysics.EngSpd[rad/s]
  __TDD__EngSpd[rad/s] : Demux  Outputs=1
  __TDD__Gear[-4;20] : Demux  Outputs=1
  Gear[-4;20] : Outport  Description=|  VectorParamsAs1DForOutWhenUnconnected=off
      | <name>DrivetrainPhysics.Transmission.Gear[-4;20]</name>
      | <comment></comment>
  EngSpd[rad/s] : Outport  Description=|  Port=2  VectorParamsAs1DForOutWhenUnconnected=off
      | <name>DrivetrainPhysics.EngSpd[rad/s]</name>
      | <comment></comment>
  wires:
  __TDD__EngSpd[rad/s]/1 -> EngSpd[rad/s]/1  "EngSpd[rad/s]"
  __TDD__Gear[-4;20]/1 -> Gear[-4;20]/1  "Gear[-4;20]"
  TDBusSelector/2 -> __TDD__EngSpd[rad/s]/1  "<EngSpd[rad/s]>"
  TDBusSelector/1 -> __TDD__Gear[-4;20]/1  "<Gear[-4;20]>"
  fromDrivetrain/1 -> TDBusSelector/1

== system SingleTrackCANoe/SimulationModel/Vehicle/Engine/EngineControlUnit/InputFromEnginePhysics ==
  fromEnginePhysics : Inport
  TDBusSelector : BusSelector  OutputSignals=Mechanics.EngTrq[Nm],Mechanics.UnrestrictedEngTrq[Nm],Mechanics.MeanEngFrictionTrq[Nm],Mechanics.MeanEngMaxTrq[Nm]
  __TDD__EngTrq[Nm] : Demux  Outputs=[1]
  __TDD__MeanEngFrictionTrq[Nm] : Demux  Outputs=1
  __TDD__MeanEngMaxTrq[Nm] : Demux  Outputs=1
  __TDD__UnrestrictedEngTrq[Nm] : Demux  Outputs=[1]
  EngTrq[Nm]___UNIQUE_1 : Outport  Description=|  PortDimensions=[1]  VectorParamsAs1DForOutWhenUnconnected=off
      | <name>Mechanics.EngTrq[Nm]</name>
      | <comment>Engine torque</comment>
  UnrestrictedEngTrq[Nm]___UNIQUE_1 : Outport  Description=|  Port=2  PortDimensions=[1]  VectorParamsAs1DForOutWhenUnconnected=off
      | <name>Mechanics.UnrestrictedEngTrq[Nm]</name>
      | <comment>Unrestricted engine torque</comment>
  MeanEngFrictionTrq[Nm]___UNIQUE_1 : Outport  Description=|  Port=3  VectorParamsAs1DForOutWhenUnconnected=off
      | <name>Mechanics.MeanEngFrictionTrq[Nm]</name>
      | <comment></comment>
  MeanEngMaxTrq[Nm]___UNIQUE_1 : Outport  Description=|  Port=4  VectorParamsAs1DForOutWhenUnconnected=off
      | <name>Mechanics.MeanEngMaxTrq[Nm]</name>
      | <comment></comment>
  wires:
  __TDD__MeanEngMaxTrq[Nm]/1 -> MeanEngMaxTrq[Nm]___UNIQUE_1/1  "MeanEngMaxTrq[Nm]"
  __TDD__MeanEngFrictionTrq[Nm]/1 -> MeanEngFrictionTrq[Nm]___UNIQUE_1/1  "MeanEngFrictionTrq[Nm]"
  __TDD__UnrestrictedEngTrq[Nm]/1 -> UnrestrictedEngTrq[Nm]___UNIQUE_1/1  "UnrestrictedEngTrq[Nm]"
  __TDD__EngTrq[Nm]/1 -> EngTrq[Nm]___UNIQUE_1/1  "EngTrq[Nm]"
  TDBusSelector/4 -> __TDD__MeanEngMaxTrq[Nm]/1  "<MeanEngMaxTrq[Nm]>"
  TDBusSelector/3 -> __TDD__MeanEngFrictionTrq[Nm]/1  "<MeanEngFrictionTrq[Nm]>"
  TDBusSelector/2 -> __TDD__UnrestrictedEngTrq[Nm]/1  "<UnrestrictedEngTrq[Nm]>"
  TDBusSelector/1 -> __TDD__EngTrq[Nm]/1  "<EngTrq[Nm]>"
  fromEnginePhysics/1 -> TDBusSelector/1

== system SingleTrackCANoe/SimulationModel/Vehicle/Engine/EnginePhysics/DynaComponentInfo ==

== system SingleTrackCANoe/SimulationModel/Vehicle/Engine/EnginePhysics/EnginePhysicsOutput ==
  Mechanics___UNIQUE_1 : Inport  Description=|
      | <name>Mechanics</name>
      | <comment></comment>
  ValidityStatus___UNIQUE_1 : Inport  Description=|  Port=2
      | <name>ValidityStatus</name>
      | <comment></comment>
  FuelSystem___UNIQUE_1 : Inport  Description=|  Port=3
      | <name>FuelSystem</name>
      | <comment></comment>
  __TDO__EnginePhysics : BusCreator  Inputs=3
  EnginePhysics___UNIQUE_1 : Outport  Description=|  VectorParamsAs1DForOutWhenUnconnected=off
      | <name>Mechanics</name>
      | <comment></comment>
  wires:
  __TDO__EnginePhysics/1 -> EnginePhysics___UNIQUE_1/1  "EnginePhysics"
  FuelSystem___UNIQUE_1/1 -> __TDO__EnginePhysics/3  "FuelSystem"
  ValidityStatus___UNIQUE_1/1 -> __TDO__EnginePhysics/2  "ValidityStatus"
  Mechanics___UNIQUE_1/1 -> __TDO__EnginePhysics/1  "Mechanics"

== system SingleTrackCANoe/SimulationModel/Vehicle/Engine/EnginePhysics/FuelSystemOutput ==
  FuelMassFlow[kg/s]___UNIQUE_1 : Inport  Description=|  PortDimensions=[1]
      | <name>FuelMassFlow[kg/s]</name>
      | <comment></comment>
  FuelMass[kg]___UNIQUE_1 : Inport  Description=|  Port=2  PortDimensions=[1]
      | <name>FuelMass[kg]</name>
      | <comment></comment>
  CurrFuelConsumEu[l/100km]___UNIQUE_1 : Inport  Description=|  Port=3  PortDimensions=[1]
      | <name>CurrFuelConsumEu[l/100km]</name>
      | <comment></comment>
  CurrFuelConsumUs[mpg]___UNIQUE_1 : Inport  Description=|  Port=4  PortDimensions=[1]
      | <name>CurrFuelConsumUs[mpg]</name>
      | <comment></comment>
  AvgFuelConsumEu[l/100km]___UNIQUE_1 : Inport  Description=|  Port=5  PortDimensions=[1]
      | <name>AvgFuelConsumEu[l/100km]</name>
      | <comment></comment>
  AvgFuelConsumUs[mpg]___UNIQUE_1 : Inport  Description=|  Port=6  PortDimensions=[1]
      | <name>AvgFuelConsumUs[mpg]</name>
      | <comment></comment>
  Efficiency[-]___UNIQUE_1 : Inport  Description=|  Port=7  PortDimensions=[1]
      | <name>Efficiency[-]</name>
      | <comment></comment>
  FuelDensity[kg/m**3]___UNIQUE_1 : Inport  Description=|  Port=8  PortDimensions=[1]
      | <name>FuelDensity[kg/m**3]</name>
      | <comment></comment>
  __TDD__FuelSystem.AvgFuelConsumEu[l/100km] : Demux  Outputs=[1]
  __TDD__FuelSystem.AvgFuelConsumUs[mpg] : Demux  Outputs=[1]
  __TDD__FuelSystem.CurrFuelConsumEu[l/100km] : Demux  Outputs=[1]
  __TDD__FuelSystem.CurrFuelConsumUs[mpg] : Demux  Outputs=[1]
  __TDD__FuelSystem.Efficiency[-] : Demux  Outputs=[1]
  __TDD__FuelSystem.FuelDensity[kg/m**3] : Demux  Outputs=[1]
  __TDD__FuelSystem.FuelMassFlow[kg/s] : Demux  Outputs=[1]
  __TDD__FuelSystem.FuelMass[kg] : Demux  Outputs=[1]
  __TDO__FuelSystem : BusCreator  Inputs=8
  FuelSystem___UNIQUE_1 : Outport  Description=|  PortDimensions=[8]  VectorParamsAs1DForOutWhenUnconnected=off
      | <name>FuelMassFlow[kg/s]</name>
      | <comment></comment>
  wires:
  __TDO__FuelSystem/1 -> FuelSystem___UNIQUE_1/1  "FuelSystem"
  __TDD__FuelSystem.FuelDensity[kg/m**3]/1 -> __TDO__FuelSystem/8  "FuelDensity[kg/m**3]"
  FuelDensity[kg/m**3]___UNIQUE_1/1 -> __TDD__FuelSystem.FuelDensity[kg/m**3]/1
  __TDD__FuelSystem.Efficiency[-]/1 -> __TDO__FuelSystem/7  "Efficiency[-]"
  Efficiency[-]___UNIQUE_1/1 -> __TDD__FuelSystem.Efficiency[-]/1
  __TDD__FuelSystem.AvgFuelConsumUs[mpg]/1 -> __TDO__FuelSystem/6  "AvgFuelConsumUs[mpg]"
  AvgFuelConsumUs[mpg]___UNIQUE_1/1 -> __TDD__FuelSystem.AvgFuelConsumUs[mpg]/1
  __TDD__FuelSystem.AvgFuelConsumEu[l/100km]/1 -> __TDO__FuelSystem/5  "AvgFuelConsumEu[l/100km]"
  AvgFuelConsumEu[l/100km]___UNIQUE_1/1 -> __TDD__FuelSystem.AvgFuelConsumEu[l/100km]/1
  __TDD__FuelSystem.CurrFuelConsumUs[mpg]/1 -> __TDO__FuelSystem/4  "CurrFuelConsumUs[mpg]"
  CurrFuelConsumUs[mpg]___UNIQUE_1/1 -> __TDD__FuelSystem.CurrFuelConsumUs[mpg]/1
  __TDD__FuelSystem.CurrFuelConsumEu[l/100km]/1 -> __TDO__FuelSystem/3  "CurrFuelConsumEu[l/100km]"
  CurrFuelConsumEu[l/100km]___UNIQUE_1/1 -> __TDD__FuelSystem.CurrFuelConsumEu[l/100km]/1
  __TDD__FuelSystem.FuelMass[kg]/1 -> __TDO__FuelSystem/2  "FuelMass[kg]"
  FuelMass[kg]___UNIQUE_1/1 -> __TDD__FuelSystem.FuelMass[kg]/1
  __TDD__FuelSystem.FuelMassFlow[kg/s]/1 -> __TDO__FuelSystem/1  "FuelMassFlow[kg/s]"
  FuelMassFlow[kg/s]___UNIQUE_1/1 -> __TDD__FuelSystem.FuelMassFlow[kg/s]/1

== system SingleTrackCANoe/SimulationModel/Vehicle/Engine/EnginePhysics/InputFromChassis ==
  fromChassis : Inport
  TDBusSelector : BusSelector  OutputSignals=VehicleBody.AbsVel[m/s]
  __TDD__AbsVel[m/s] : Demux  Outputs=1
  AbsVel[m/s]___UNIQUE_1 : Outport  Description=|  VectorParamsAs1DForOutWhenUnconnected=off
      | <name>VehicleBody.AbsVel[m/s]</name>
      | <comment></comment>
  wires:
  __TDD__AbsVel[m/s]/1 -> AbsVel[m/s]___UNIQUE_1/1  "AbsVel[m/s]"
  TDBusSelector/1 -> __TDD__AbsVel[m/s]/1  "<AbsVel[m/s]>"
  fromChassis/1 -> TDBusSelector/1

== system SingleTrackCANoe/SimulationModel/Vehicle/Engine/EnginePhysics/InputFromDrivetrain ==
  fromDrivetrain : Inport
  TDBusSelector : BusSelector  OutputSignals=DrivetrainPhysics.EngSpd[rad/s]
  __TDD__EngSpd[rad/s] : Demux  Outputs=1
  EngSpd[rad/s] : Outport  Description=|  VectorParamsAs1DForOutWhenUnconnected=off
      | <name>DrivetrainPhysics.EngSpd[rad/s]</name>
      | <comment></comment>
  wires:
  __TDD__EngSpd[rad/s]/1 -> EngSpd[rad/s]/1  "EngSpd[rad/s]"
  TDBusSelector/1 -> __TDD__EngSpd[rad/s]/1  "<EngSpd[rad/s]>"
  fromDrivetrain/1 -> TDBusSelector/1
